simulink model "Parameter_Estimation_SM_Model_tutorial_R2018II"  (R2018a)
settings: Solver=VariableStepAuto  StartTime=0.0  StopTime=150  RelTol=1e-3
values from neighbouring files (symbols this model uses):
  D = 1.5e-3    (= 0.0015)    [initial_consts_tutorial.m]    (also in matlab.mat; matlab_final.mat = 0.0122430626368)
  Gear_Ratio = 1    [initial_consts_tutorial.m]    (also in matlab.mat; matlab_final.mat)
  J = 9.31e-4    (= 0.000931)    [initial_consts_tutorial.m]    (also in matlab.mat; matlab_final.mat = 0.00138961338286)
  Kb = 0.00767    [initial_consts_tutorial.m]    (also in matlab.mat; matlab_final.mat = -0.0590015655032)
  Kt = 0.00767    [initial_consts_tutorial.m]    (also in matlab.mat; matlab_final.mat = -0.0565055058784)
  L = 0.001    [initial_consts_tutorial.m]    (also in matlab.mat; matlab_final.mat = 0.0195332969567)
  R = 2.6    [initial_consts_tutorial.m]    (also in matlab.mat; matlab_final.mat = 4.44397012968)
undefined symbols (not defined in the file or in its folder): sigbuilder_block
settings Model: OrderedModelArguments=off  Creator=Ahmed  LastModifiedBy=PC
settings DataIOCC: ReturnWorkspaceOutputs=on
settings SFSimCC: SimUseLocalCustomCode=on
settings RTWCC: RTWUseLocalCustomCode=on

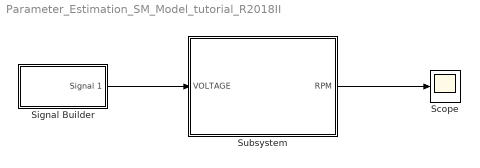
== system Parameter_Estimation_SM_Model_tutorial_R2018II ==
  Scope : Scope
  Signal Builder : Subsystem  Tag=STV Subsys  LoadFcn=sigbuilder_block('load');  StartFcn=sigbuilder_block('start');  StopFcn=sigbuilder_block('stop');  ClipboardFcn=sigbuilder_block('clipboard');  mask(Sigbuilder block){tuvar=[0:10]}
      mask help: Simulink:masks:SigbuilderBlock_MD
      mask init:
      | if ~strcmp(get_param(bdroot(gcbh),'SimulationStatus'),'stopped') tuvar = sigbuilder_block('maskInit'); end
      settings: CopyFcn=sigbuilder_block('copy');  DeleteFcn=sigbuilder_block('delete');  ModelCloseFcn=sigbuilder_block('modelClose');  PreSaveFcn=sigbuilder_block('preSave');  PauseFcn=sigbuilder_block('pause');  ContinueFcn=sigbuilder_block('continue');  NameChangeFcn=sigbuilder_block('namechange');  OpenFcn=sigbuilder_block('open',[251.4 72.6 550.2 418.2 ]);  CloseFcn=sigbuilder_block('close');
      mask Display: plot(0, 0, 100, 100,[2, 2, 32, 32, 2], [68, 8, 8, 68, 68],[32, 2], [38, 38], [32, 19, 2],[53, 60, 44], [32, 17, 17, 2],[16, 16, 31, 31]);txt = getActiveGroup(gcbh);text(2, 100, txt,'verticalAlignment', 'top');
  Subsystem : Subsystem
      mask Display:
      | color ('red')
      | port_label('input',1,'V')
      | color ('blue')
      | port_label('output',1,'RPM')
  wires:
  Subsystem/1(RPM) -> Scope/1
  Signal Builder/1(Signal 1) -> Subsystem/1(VOLTAGE)

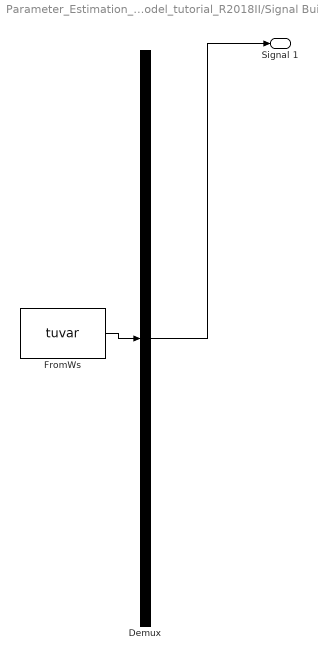
== system Parameter_Estimation_SM_Model_tutorial_R2018II/Signal Builder ==
  Demux : Demux  Tag=STV Demux  Outputs=1
  FromWs : FromWorkspace  Tag=STV FromWs  VariableName=tuvar  SampleTime=0
      SigBuilderData=|
      | common.afterFinalStr = 'Extrapolate'
      | common.sampleTime = 0
      | dataSet.timeRange = [0 150]
      | dataSet.name = 'Group 1'
      | sbobj.Groups.Name = 'Group 1'
      | sbobj.Groups.Signals.Name = 'Signal 1'
      | sbobj.Groups.Signals.XData = [0 0.1 0.2 0.3 0.4 0.5 0.6 0.7 0.8 0.9 1 1.1 ... (1151 elements, 1x1151)]
      | sbobj.Groups.Signals.YData = [0 0 0 0 0 0 0 0 0 0 0 0 ... (1151 elements, 1x1151)]
      | sbobj.Groups.TimeRange = [0 150]
  Signal 1 : Outport  Tag=STV Outport  VectorParamsAs1DForOutWhenUnconnected=on
  wires:
  FromWs/1 -> Demux/1
  Demux/1 -> Signal 1/1

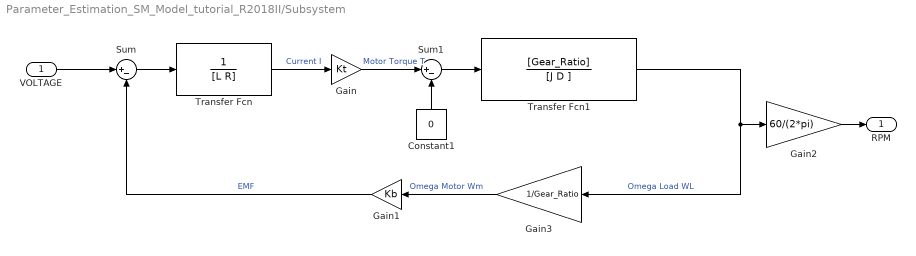
== system Parameter_Estimation_SM_Model_tutorial_R2018II/Subsystem ==
  VOLTAGE : Inport
  Constant1 : Constant  Value=0
  Gain : Gain  Gain=Kt
  Gain1 : Gain  Gain=Kb
  Gain2 : Gain  Gain=60/(2*pi)
  Gain3 : Gain  Gain=1/Gear_Ratio
  Sum : Sum  Inputs=|+-
  Sum1 : Sum  Inputs=|+-
  Transfer Fcn : TransferFcn  Denominator=[L R]
  Transfer Fcn1 : TransferFcn  Numerator=[Gear_Ratio]  Denominator=[J D ]
  RPM : Outport  VectorParamsAs1DForOutWhenUnconnected=on
  wires:
  Transfer Fcn1/1 -> Gain2/1, Gain3/1  "Omega Load WL"
  Transfer Fcn/1 -> Gain/1  "Current I"
  Gain/1 -> Sum1/1  "Motor Torque T"
  Sum/1 -> Transfer Fcn/1
  Sum1/1 -> Transfer Fcn1/1
  Constant1/1 -> Sum1/2
  Gain1/1 -> Sum/2  "EMF"
  VOLTAGE/1 -> Sum/1
  Gain2/1 -> RPM/1
  Gain3/1 -> Gain1/1  "Omega Motor Wm"
